simulink model "TV_2018_HIL"  (R2016a)
settings: Solver=FixedStepAuto  StartTime=0.0  StopTime=inf  FixedStep=0.001  RelTol=1e-3
PreLoadFcn:
  | TV_2017_parameters
values from neighbouring files (symbols this model uses):
  battery_voltage = single(530)    [HIL_parameters.m]    (also in HIL_parameters_2018.m; TV_2017_parameters.m; TV_2017_parameters_VD.m)
  car_params = Simulink_Car_params    [HIL_parameters.m]    (also in HIL_parameters_2018.m; TV_2017_parameters.m; TV_2017_parameters_VD.m)
  i_Diff = 16    [HIL_parameters.m]    (also in HIL_parameters_2018.m; TV_2017_parameters.m)
  Kp = 1    [HIL_parameters.m]    (also in HIL_parameters_2018.m; TV_2017_parameters.m; TV_2017_parameters_VD.m)
  motor_data = struct    [HIL_parameters.m]    (also in HIL_parameters_2018.m; TV_2017_parameters.m)
  powerLimitControl = Simulink_el    [HIL_parameters.m]    (also in HIL_parameters_2018.m; TV_2017_parameters.m; TV_2017_parameters_VD.m)
  settings = Simulink_Settings    [HIL_parameters.m]    (also in HIL_parameters_2018.m; TV_2017_parameters.m; TV_2017_parameters_VD.m)
  SpdC_BCC = 0    [HIL_parameters.m]    (also in HIL_parameters_2018.m; TV_2017_parameters.m; TV_2017_parameters_VD.m)
  Speed_Neg_sat = -21    [HIL_parameters.m]    (also in HIL_parameters_2018.m; TV_2017_parameters.m; TV_2017_parameters_VD.m)
  Speed_Pos_sat = 21    [HIL_parameters.m]    (also in HIL_parameters_2018.m; TV_2017_parameters.m; TV_2017_parameters_VD.m)
  SteeringAngleFL = [-23.80 -22.65 -21.50 -20.34 -19.18 -18.03 -16.86 -15.70 -14.53 -13.35 -12.18 -10.99 -9.80 -8.61 -7.40 -6.19 -4.97 -3.75 -2.51 -1.26 0 1.27 2.56 3.85 5.17 6.50 7.84 9.21 10.59 12.00 13.42 14.88 16.36 17.87 19.41 20.99 22.61 24.26 25.97 27.73 29.54]    [CarSetupAnalysis2018.m]    (also in HIL_parameters_2018.m; TV_2017_parameters.m; TV_2017_parameters_VD.m = [-24.129 -22.950 -21.772 -20.593 -19.413 -18.232 -17.050 -15)
  SteeringAngleFR = [-29.54 -27.73 -25.97 -24.26 -22.61 -20.99 -19.41 -17.87 -16.36 -14.88 -13.42 -12.00 -10.59 -9.21 -7.84 -6.50 -5.17 -3.85 -2.56 -1.27 0 1.26 2.51 3.75 4.97 6.19 7.40 8.61 9.80 10.99 12.18 13.35 14.53 15.70 16.86 18.03 19.18 20.34 21.50 22.65 23.80]    [CarSetupAnalysis2018.m]    (also in HIL_parameters_2018.m; TV_2017_parameters.m; TV_2017_parameters_VD.m = [-29.3050 -27.5340 -25.8140 -24.1410 -22.5110 -20.9180 -19.3)
  SteeringWhAngle = [-105 -99.75 -94.5 -89.25 -84 -78.75 -73.5 -68.25 -63 -57.75 -52.5 -47.25 -42 -36.75 -31.5 -26.25 -21.0 -15.75 -10.5 -5.25 0.0 5.25 10.50 15.75 21.00 26.25 31.50 36.75 42.00 47.25 52.50 57.75  63.00 68.25 73.50 78.75 84.00 89.25 94.50 99.75 105.00]    [TV_2017_parameters_VD.m]
  Tn_n = 0    [HIL_parameters.m]    (also in HIL_parameters_2018.m; TV_2017_parameters.m; TV_2017_parameters_VD.m)
  tractionControl = Simulink_tc    [HIL_parameters.m]    (also in HIL_parameters_2018.m; IterativeTractionControlTuning.m; TV_2017_parameters.m; TV_2017_parameters_VD.m)
  yawMomentGenerator = struct    [HIL_parameters.m]    (also in HIL_parameters_2018.m = Simulink_yawRate2; TV_2017_parameters.m = Simulink_yawRate2)
  yawRateControl = Simulink_yawRate    [HIL_parameters.m]    (also in HIL_parameters_2018.m; TV_2017_parameters.m; TV_2017_parameters_VD.m)
undefined symbols (not defined in the file or in its folder): canChannel, DiscIntNeverNeededParam, magnitude, speedEstimation, TC_Decr_Gas, TC_Derivative, TC_Incr_Gas, TC_On, TC_Relay_Off, TC_Relay_On
libraries: CarMaker4SL x366, simulink_extras x63, canmsglib x55, canlib x41, simulink x37, dspfdesign x2, sldrtlib x1
(part 5 of 15)

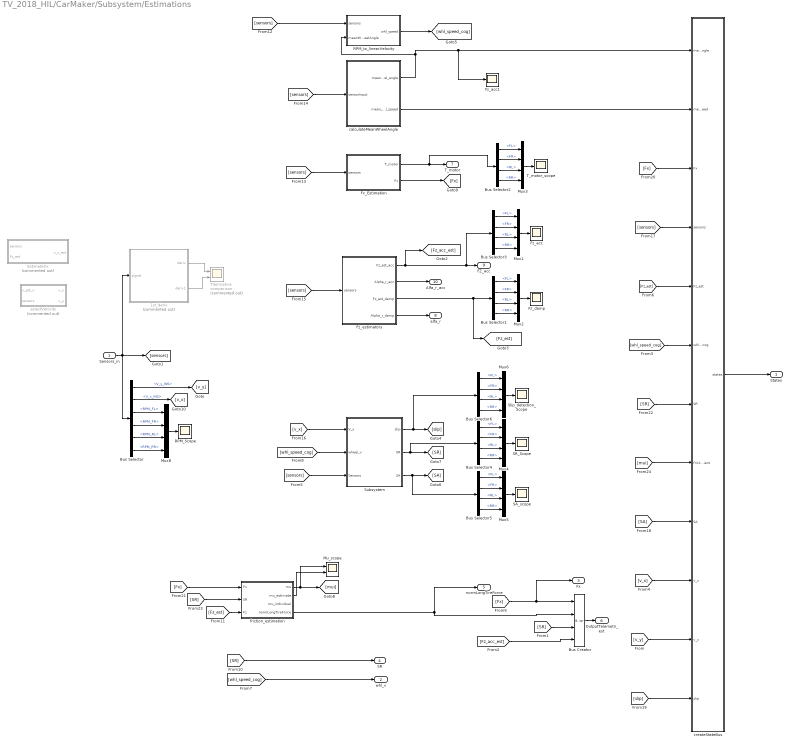
== system TV_2018_HIL/CarMaker/Subsystem/Estimations ==
  Sensors_in : Inport
  1st_deriv : Subsystem  Commented=on
  Bus Creator : BusCreator  Inputs=4  OutDataTypeStr=Bus: OutputTelemetri_est
      settings: InheritFromInputs=off
  Bus Selector : BusSelector  OutputSignals=V_y_INS,V_x_INS,RPM_FL,RPM_FR,RPM_RL,RPM_RR
  Bus Selector{1..6} (6 alike) : BusSelector  OutputSignals=FL,FR,RL,RR
  EstimateVx : Subsystem  Commented=on
  Fx_Estimation : Subsystem
  Fz_acc : Scope
  Fz_acc1 : Scope
  Fz_damp : Scope
  Fz_estimators : Subsystem
  Mu_scope : Scope  NumInputPorts=2
  Mux{1..6,8} (7 alike) : Mux
  RPM_Scope : Scope
  RPM_to_linearVelocity : Subsystem
  SA_scope : Scope
  SR_Scope : Scope
  Slip_detection_Scope : Scope
  Subsystem : Subsystem
  T_motor_scope : Scope
  Tderivative comparison : Scope  Commented=on  NumInputPorts=2
  calculateMeanWheelAngle : Subsystem
  createStateBus : Subsystem
  friction_estimation : Subsystem
  selectVelocity : Subsystem  Commented=on
  States : Outport
  whl_v : Outport  Port=2
  Fx : Outport  Port=3
  SR : Outport  Port=4
  normLongTireForce : Outport  Port=5
  OutputTelemetri_est : Outport  Port=6
  T_motor : Outport  Port=7
  alfa_r : Outport  Port=8
  FZ_acc : Outport  Port=9
  "Alfa_r_acc " : Outport  Port=10
  wires:
  Fx_Estimation/2(Fx) -> [Fx]
  RPM_to_linearVelocity/1(whl_speed) -> [whl_speed_cog]
  createStateBus/1(states) -> States/1
  [v_y] -> createStateBus/11(v_y)
  [v_x] -> createStateBus/10(v_x)
  [whl_speed_cog] -> createStateBus/6(whl_speed_cog)
  friction_estimation/1(mu) -> [mui], Mu_scope/1
  [whl_speed_cog] -> whl_v/1
  [Fx] -> Bus Creator/1, Fx/1
  [SR] -> SR/1
  friction_estimation/4(normLongTireForce) -> normLongTireForce/1, Bus Creator/2
  Bus Creator/1 -> OutputTelemetri_est/1
  [Fz_est] -> friction_estimation/3(Fz)
  calculateMeanWheelAngle/1(mean_wheel_angle) -> Fz_acc1/1, createStateBus/1(mean_wheel_angle), RPM_to_linearVelocity/2(meanWheelAngle)
  calculateMeanWheelAngle/2(mean_wheel_speed) -> createStateBus/2(mean_wheel_speed)
  Fx_Estimation/1(T_motor) -> Bus Selector2/1, T_motor/1
  Sensors_in/1 -> Bus Selector/1, [sensors], 1st_deriv/1(signal)
  [sensors] -> RPM_to_linearVelocity/1(sensors)
  [sensors] -> Fx_Estimation/1(sensors)
  [sensors] -> calculateMeanWheelAngle/1(sensorInput)
  [sensors] -> createStateBus/4(sensors)
  Bus Selector/2 -> [v_x]  "<V_x_INS>"
  Bus Selector/1 -> [v_y]  "<V_y_INS>"
  [SR] -> Bus Creator/3
  [Fz_acc_est] -> Bus Creator/4
  [Fz_est] -> createStateBus/5(Fz_est)
  [Fx] -> createStateBus/3(Fx)
  [Fx] -> friction_estimation/1(Fx)
  [SR] -> createStateBus/7(SR)
  [SR] -> friction_estimation/2(SR)
  [mui] -> createStateBus/8(frictionCoefficient)
  Bus Selector3/1 -> Mux1/1  "<FL>"
  Bus Selector3/2 -> Mux1/2  "<FR>"
  Bus Selector3/3 -> Mux1/3  "<RL>"
  Bus Selector3/4 -> Mux1/4  "<RR>"
  Mux1/1 -> Fz_acc/1
  Bus Selector1/1 -> Mux2/1  "<FL>"
  Bus Selector1/2 -> Mux2/2  "<FR>"
  Bus Selector1/3 -> Mux2/3  "<RL>"
  Bus Selector1/4 -> Mux2/4  "<RR>"
  Mux2/1 -> Fz_damp/1
  Bus Selector2/1 -> Mux3/1  "<FL>"
  Bus Selector2/2 -> Mux3/2  "<FR>"
  Bus Selector2/3 -> Mux3/3  "<RL>"
  Bus Selector2/4 -> Mux3/4  "<RR>"
  Mux3/1 -> T_motor_scope/1
  Bus Selector4/1 -> Mux4/1  "<FL>"
  Bus Selector4/2 -> Mux4/2  "<FR>"
  Bus Selector4/3 -> Mux4/3  "<RL>"
  Bus Selector4/4 -> Mux4/4  "<RR>"
  Mux4/1 -> SR_Scope/1
  1st_deriv/1(deriv) -> Tderivative comparison/1
  1st_deriv/2(deriv1) -> Tderivative comparison/2
  friction_estimation/2(mu_estimate) -> Mu_scope/2
  Bus Selector5/1 -> Mux5/1  "<FL>"
  Bus Selector5/2 -> Mux5/2  "<FR>"
  Bus Selector5/3 -> Mux5/3  "<RL>"
  Bus Selector5/4 -> Mux5/4  "<RR>"
  Mux5/1 -> SA_scope/1
  Bus Selector6/1 -> Mux6/1  "<FL>"
  Bus Selector6/2 -> Mux6/2  "<FR>"
  Bus Selector6/3 -> Mux6/3  "<RL>"
  Bus Selector6/4 -> Mux6/4  "<RR>"
  Mux6/1 -> Slip_detection_Scope/1
  Fz_estimators/3(Fz_est_damp) -> Bus Selector1/1, [Fz_est]
  Fz_estimators/1(Fz_est_acc) -> [Fz_acc_est], Bus Selector3/1, FZ_acc/1
  [sensors] -> Fz_estimators/1(sensors)
  Fz_estimators/2(Alpha_r_acc) -> "Alfa_r_acc "/1
  Fz_estimators/4(Alpha_r_damp) -> alfa_r/1
  [v_x] -> Subsystem/1(V_x)
  [whl_speed_cog] -> Subsystem/2(wheel_v)
  [sensors] -> Subsystem/3(Sensors)
  Subsystem/1(slip) -> Bus Selector6/1, [slip]
  Subsystem/2(SR) -> Bus Selector4/1, [SR]
  [SA] -> createStateBus/9(SA)
  Subsystem/3(SA) -> Bus Selector5/1, [SA]
  [slip] -> createStateBus/12(slip)
  Mux8/1 -> RPM_Scope/1
  Bus Selector/3 -> Mux8/1  "<RPM_FL>"
  Bus Selector/4 -> Mux8/2  "<RPM_FR>"
  Bus Selector/5 -> Mux8/3  "<RPM_RL>"
  Bus Selector/6 -> Mux8/4  "<RPM_RR>"

== system TV_2018_HIL/CarMaker/VehicleControl3/CreateBus Vhcl.Misc ==
  In1 : Inport
  BusCreator : BusCreator  Inputs=11
  Demux : Demux  Outputs=11
  Out1 : Outport
  wires:
  Demux/11 -> BusCreator/11  "Vhcl Wind_vel_0 z"
  Demux/10 -> BusCreator/10  "Vhcl Wind_vel_0 y"
  Demux/9 -> BusCreator/9  "Vhcl Wind_vel_0 x"
  Demux/8 -> BusCreator/8  "Vhcl Trq_DL2BdyEng y"
  Demux/7 -> BusCreator/7  "Vhcl Trq_DL2BdyEng x"
  Demux/6 -> BusCreator/6  "Vhcl Trq_DL2Bdy1B z"
  Demux/5 -> BusCreator/5  "Vhcl Trq_DL2Bdy1B y"
  Demux/4 -> BusCreator/4  "Vhcl Trq_DL2Bdy1B x"
  Demux/3 -> BusCreator/3  "Vhcl Trq_DL2Bdy1 z"
  Demux/2 -> BusCreator/2  "Vhcl Trq_DL2Bdy1 y"
  Demux/1 -> BusCreator/1  "Vhcl Trq_DL2Bdy1 x"
  In1/1 -> Demux/1
  BusCreator/1 -> Out1/1

== system TV_2018_HIL/CarMaker/VehicleControl3/CreateBus Vhcl.Wheel.In ==
  In1 : Inport
  Bus Creator1 : BusCreator  Inputs=12
  Demux1 : Demux  Outputs=12
  Out1 : Outport
  wires:
  Demux1/12 -> Bus Creator1/12  "Vhcl Wheel RR rotv"
  Demux1/11 -> Bus Creator1/11  "Vhcl Wheel RR Trq_DL2WC"
  Demux1/10 -> Bus Creator1/10  "Vhcl Wheel RR Trq_B2WC"
  Demux1/9 -> Bus Creator1/9  "Vhcl Wheel RL rotv"
  Demux1/8 -> Bus Creator1/8  "Vhcl Wheel RL Trq_DL2WC"
  Demux1/7 -> Bus Creator1/7  "Vhcl Wheel RL Trq_B2WC"
  Demux1/6 -> Bus Creator1/6  "Vhcl Wheel FR rotv"
  Demux1/5 -> Bus Creator1/5  "Vhcl Wheel FR Trq_DL2WC"
  Demux1/4 -> Bus Creator1/4  "Vhcl Wheel FR Trq_B2WC"
  Demux1/3 -> Bus Creator1/3  "Vhcl Wheel FL rotv"
  In1/1 -> Demux1/1
  Bus Creator1/1 -> Out1/1
  Demux1/2 -> Bus Creator1/2  "Vhcl Wheel FL Trq_DL2WC"
  Demux1/1 -> Bus Creator1/1  "Vhcl Wheel FL Trq_B2WC"

== system TV_2018_HIL/CarMaker/VehicleControl3/CreateBus VhclCtrl ==
  In : Inport
  BusCreator : BusCreator  Inputs=29
  Demux : Demux  Outputs=29
  Out : Outport
  wires:
  In/1 -> Demux/1
  BusCreator/1 -> Out/1
  Demux/1 -> BusCreator/1  "VhclCtrl SST"
  Demux/2 -> BusCreator/2  "VhclCtrl Key"
  Demux/3 -> BusCreator/3  "VhclCtrl UserSignal0"
  Demux/4 -> BusCreator/4  "VhclCtrl UserSignal1"
  Demux/5 -> BusCreator/5  "VhclCtrl UserSignal2"
  Demux/6 -> BusCreator/6  "VhclCtrl UserSignal3"
  Demux/7 -> BusCreator/7  "VhclCtrl UserSignal4"
  Demux/8 -> BusCreator/8  "VhclCtrl GearNo"
  Demux/9 -> BusCreator/9  "VhclCtrl SelectorCtrl"
  Demux/10 -> BusCreator/10  "VhclCtrl Brake"
  Demux/11 -> BusCreator/11  "VhclCtrl BrakePark"
  Demux/12 -> BusCreator/12  "VhclCtrl Clutch"
  Demux/13 -> BusCreator/13  "VhclCtrl Gas"
  Demux/14 -> BusCreator/14  "VhclCtrl Steering Ang"
  Demux/15 -> BusCreator/15  "VhclCtrl Steering AngVel"
  Demux/16 -> BusCreator/16  "VhclCtrl Steering AngAcc"
  Demux/17 -> BusCreator/17  "VhclCtrl Steering Trq"
  Demux/18 -> BusCreator/18  "VhclCtrl Lights LowBeam"
  Demux/19 -> BusCreator/19  "VhclCtrl Lights HighBeam"
  Demux/20 -> BusCreator/20  "VhclCtrl Lights Daytime"
  Demux/21 -> BusCreator/21  "VhclCtrl Lights ParkL"
  Demux/22 -> BusCreator/22  "VhclCtrl Lights ParkR"
  Demux/23 -> BusCreator/23  "VhclCtrl Lights IndL"
  Demux/24 -> BusCreator/24  "VhclCtrl Lights IndR"
  Demux/25 -> BusCreator/25  "VhclCtrl Lights FogFrontL"
  Demux/26 -> BusCreator/26  "VhclCtrl Lights FogFrontR"
  Demux/27 -> BusCreator/27  "VhclCtrl Lights FogRear"
  Demux/28 -> BusCreator/28  "VhclCtrl Lights Brake"
  Demux/29 -> BusCreator/29  "VhclCtrl Lights Reverse"

== system TV_2018_HIL/CarMaker/VehicleControl3/CreateBus VhclCtrl.PT ==
  In1 : Inport
  BusCreator1 : BusCreator  Inputs=12
  Demux1 : Demux  Outputs=12
  Out1 : Outport
  wires:
  Demux1/12 -> BusCreator1/12  "VhclCtrl Brake"
  Demux1/11 -> BusCreator1/11  "VhclCtrl Gas"
  Demux1/10 -> BusCreator1/10  "VhclCtrl Clutch"
  Demux1/9 -> BusCreator1/9  "VhclCtrl SelectorCtrl"
  Demux1/8 -> BusCreator1/8  "VhclCtrl GearNo"
  Demux1/7 -> BusCreator1/7  "VhclCtrl UserSignal4"
  Demux1/6 -> BusCreator1/6  "VhclCtrl UserSignal3"
  Demux1/5 -> BusCreator1/5  "VhclCtrl UserSignal2"
  Demux1/4 -> BusCreator1/4  "VhclCtrl UserSignal1"
  Demux1/3 -> BusCreator1/3  "VhclCtrl UserSignal0"
  Demux1/2 -> BusCreator1/2  "VhclCtrl Key"
  Demux1/1 -> BusCreator1/1  "VhclCtrl SST"
  In1/1 -> Demux1/1
  BusCreator1/1 -> Out1/1

== system TV_2018_HIL/CarMaker/VehicleControl3/CreateBus VhclCtrl.Steering ==
  In1 : Inport
  Bus Creator : BusCreator  Inputs=5
  Demux : Demux  Outputs=5
  Out1 : Outport
  wires:
  In1/1 -> Demux/1
  Bus Creator/1 -> Out1/1
  Demux/1 -> Bus Creator/1  "VhclCtrl Steering Ang"
  Demux/5 -> Bus Creator/5  "VhclCtrl Steering SteerByTrq"
  Demux/3 -> Bus Creator/3  "VhclCtrl Steering AngAcc"
  Demux/2 -> Bus Creator/2  "VhclCtrl Steering AngVel"
  Demux/4 -> Bus Creator/4  "VhclCtrl Steering Trq"

== system TV_2018_HIL/CarMaker/IPG Vehicle3/Brake/CreateBus Vhcl.Wheel.PT ==
  In : Inport
  BusCreator1 : BusCreator  Inputs=20
  Demux1 : Demux  Outputs=20
  Out : Outport
  wires:
  Demux1/20 -> BusCreator1/20  "Vhcl Trq_DriveSrc_trg d3"
  Demux1/19 -> BusCreator1/19  "Vhcl Trq_DriveSrc_trg d2"
  Demux1/18 -> BusCreator1/18  "Vhcl Trq_DriveSrc_trg d1"
  Demux1/17 -> BusCreator1/17  "Vhcl Trq_DriveSrc_trg d0"
  Demux1/16 -> BusCreator1/16  "Vhcl Wheel RR WhlBearing"
  Demux1/15 -> BusCreator1/15  "Vhcl Wheel RR Trq_T2W"
  Demux1/14 -> BusCreator1/14  "Vhcl Wheel RR Trq_BrakeReg_trg"
  Demux1/13 -> BusCreator1/13  "Vhcl Wheel RR Trq_Brake"
  Demux1/12 -> BusCreator1/12  "Vhcl Wheel RL WhlBearing"
  Demux1/11 -> BusCreator1/11  "Vhcl Wheel RL Trq_T2W"
  Demux1/10 -> BusCreator1/10  "Vhcl Wheel RL Trq_BrakeReg_trg"
  Demux1/9 -> BusCreator1/9  "Vhcl Wheel RL Trq_Brake"
  Demux1/8 -> BusCreator1/8  "Vhcl Wheel FR WhlBearing"
  Demux1/7 -> BusCreator1/7  "Vhcl Wheel FR Trq_T2W"
  Demux1/6 -> BusCreator1/6  "Vhcl Wheel FR Trq_BrakeReg_trg"
  Demux1/5 -> BusCreator1/5  "Vhcl Wheel FR Trq_Brake"
  Demux1/4 -> BusCreator1/4  "Vhcl Wheel FL WhlBearing"
  Demux1/3 -> BusCreator1/3  "Vhcl Wheel FL Trq_T2W"
  Demux1/2 -> BusCreator1/2  "Vhcl Wheel FL Trq_BrakeReg_trg"
  Demux1/1 -> BusCreator1/1  "Vhcl Wheel FL Trq_Brake"
  BusCreator1/1 -> Out/1
  In/1 -> Demux1/1

== system TV_2018_HIL/CarMaker/IPG Vehicle3/CarAndTrailer/CarAndTrailerUpd ==
  Sync_In : Inport
  Vhcl.Steering : Inport  Port=2
  Vhcl.Motion : Inport  Port=3
  Vhcl.PoI : Inport  Port=4
  Vhcl.Wheel.FL : Inport  Port=5
  Vhcl.Wheel.FR : Inport  Port=6
  Vhcl.Wheel.RL : Inport  Port=7
  Vhcl.Wheel.RR : Inport  Port=8
  Car.Hitch.FrcTrq : Inport  Port=9
  Vhcl.Fr1A : Inport  Port=10
  CarAndTrailerUpd : S-Function  FunctionName=CM_Sfun  Parameters='CarAndTrUpd'  SFunctionDeploymentMode=off  EnableBusSupport=off
  CreateBus Brake.IF.In : Subsystem
  Sync_Out : Outport
  Brake.IF.In : Outport  Port=2
  wires:
  Vhcl.Fr1A/1 -> CarAndTrailerUpd/10  "user vehicle only"
  Vhcl.Steering/1 -> CarAndTrailerUpd/2
  Vhcl.Motion/1 -> CarAndTrailerUpd/3
  Vhcl.PoI/1 -> CarAndTrailerUpd/4
  Vhcl.Wheel.FL/1 -> CarAndTrailerUpd/5
  Vhcl.Wheel.FR/1 -> CarAndTrailerUpd/6
  Car.Hitch.FrcTrq/1 -> CarAndTrailerUpd/9
  Vhcl.Wheel.RR/1 -> CarAndTrailerUpd/8
  Vhcl.Wheel.RL/1 -> CarAndTrailerUpd/7
  CarAndTrailerUpd/2 -> CreateBus Brake.IF.In/1(In)
  CreateBus Brake.IF.In/1(Out) -> Brake.IF.In/1
  CarAndTrailerUpd/1 -> Sync_Out/1
  Sync_In/1 -> CarAndTrailerUpd/1

== system TV_2018_HIL/CarMaker/IPG Vehicle3/CarAndTrailer/Forces ==
  Sync_In : Inport
  TireFL_In : Inport  Port=2
  TireFR_In : Inport  Port=3
  TireRL_In : Inport  Port=4
  TireRR_In : Inport  Port=5
  lSpring : Inport  Port=6
  vDamp : Inport  Port=7
  lStabi : Inport  Port=8
  lBuf : Inport  Port=9
  External Suspension Forces : Subsystem
  Tires : Subsystem
  Vehicle Forces : Subsystem
  Sync_Out : Outport
  Car.Virtual : Outport  Port=2
  Car.Aero : Outport  Port=3
  Car.Load : Outport  Port=4
  TireFL_Out : Outport  Port=5
  TireFR_Out : Outport  Port=6
  TireRL_Out : Outport  Port=7
  TireRR_Out : Outport  Port=8
  FSpring : Outport  Port=9
  FDamp : Outport  Port=10
  FStabi : Outport  Port=11
  FBuf : Outport  Port=12
  wires:
  lBuf/1 -> External Suspension Forces/5(lBuf)
  lStabi/1 -> External Suspension Forces/4(lStabi)
  vDamp/1 -> External Suspension Forces/3(vDamp)
  Tires/4(TireRR_Out) -> TireRR_Out/1
  Tires/3(TireRL_Out) -> TireRL_Out/1
  Tires/2(TireFR_Out) -> TireFR_Out/1
  Tires/1(TireFL_Out) -> TireFL_Out/1
  TireRR_In/1 -> Tires/5(TireRR_In)
  TireRL_In/1 -> Tires/4(TireRL_In)
  TireFR_In/1 -> Tires/3(TireFR_In)
  TireFL_In/1 -> Tires/2(TireFL_In)
  External Suspension Forces/4(FBuf) -> FBuf/1
  Sync_In/1 -> External Suspension Forces/1(Sync_In), Tires/1(Sync_In), Vehicle Forces/1(Sync_In)
  Vehicle Forces/1(Sync_Out) -> Sync_Out/1
  Vehicle Forces/2(Car.Virtual) -> Car.Virtual/1
  Vehicle Forces/3(Car.Aero) -> Car.Aero/1
  Vehicle Forces/4(Car.Load) -> Car.Load/1
  lSpring/1 -> External Suspension Forces/2(lSpring)
  External Suspension Forces/2(FDamp) -> FDamp/1
  External Suspension Forces/3(FStabi) -> FStabi/1
  External Suspension Forces/1(FSpring) -> FSpring/1

== system TV_2018_HIL/CarMaker/IPG Vehicle3/CarAndTrailer/Kinematics ==
  Sync_In : Inport
  Steer.IF : Inport  Port=2
  Kinematics : S-Function  FunctionName=CM_Sfun  Parameters='Kinematics'  SFunctionDeploymentMode=off  EnableBusSupport=off
  Sync_Out : Outport
  TireFL_In : Outport  Port=2
  TireFR_In : Outport  Port=3
  TireRL_In : Outport  Port=4
  TireRR_In : Outport  Port=5
  lSpring : Outport  Port=6
  vDamp : Outport  Port=7
  lStabi : Outport  Port=8
  lBuf : Outport  Port=9
  wires:
  Kinematics/9 -> lBuf/1
  Kinematics/8 -> lStabi/1
  Kinematics/2 -> TireFL_In/1
  Kinematics/3 -> TireFR_In/1
  Kinematics/4 -> TireRL_In/1
  Kinematics/5 -> TireRR_In/1
  Kinematics/6 -> lSpring/1
  Kinematics/7 -> vDamp/1
  Sync_In/1 -> Kinematics/1
  Kinematics/1 -> Sync_Out/1
  Steer.IF/1 -> Kinematics/2

== system TV_2018_HIL/CarMaker/IPG Vehicle3/CarAndTrailer/Kinetics ==
  Sync_In : Inport
  Car.Virtual : Inport  Port=2
  Car.Aero : Inport  Port=3
  Car.Load : Inport  Port=4
  TireFL.Out : Inport  Port=5
  TireFR.Out : Inport  Port=6
  TireRL.Out : Inport  Port=7
  TireRR.Out : Inport  Port=8
  FSpring : Inport  Port=9
  FDamp : Inport  Port=10
  FStabi : Inport  Port=11
  FBuf : Inport  Port=12
  Bus Creator : BusCreator  Inputs=4
  Bus Creator1 : BusCreator  Inputs=12
  Bus Creator2 : BusCreator  Inputs=6
  Bus Creator3 : BusCreator  Inputs=6
  Bus Creator4 : BusCreator  Inputs=4
  Demux : Demux  Outputs=12
  Demux1 : Demux  Outputs=6
  Demux2 : Demux  Outputs=6
  Demux3 : Demux
  Demux4 : Demux
  Kinetics : S-Function  FunctionName=CM_Sfun  Parameters='Kinetics'  SFunctionDeploymentMode=off  EnableBusSupport=off
  Sync_Out : Outport
  Trailer.Load : Outport  Port=2
  Car.Hitch : Outport  Port=3
  Car.Fr1 : Outport  Port=4
  Car.Trq_T2W : Outport  Port=5
  WheelCarrier.Misc : Outport  Port=6
  wires:
  FBuf/1 -> Kinetics/12
  Sync_In/1 -> Kinetics/1
  Kinetics/1 -> Sync_Out/1
  Car.Aero/1 -> Kinetics/3
  Car.Virtual/1 -> Kinetics/2
  Bus Creator1/1 -> Trailer.Load/1
  Demux/1 -> Bus Creator1/1  "Trailer Load_0 mass"
  Demux/2 -> Bus Creator1/2  "Trailer Load_0 tx"
  Demux/3 -> Bus Creator1/3  "Trailer Load_0 ty"
  Demux/4 -> Bus Creator1/4  "Trailer Load_0 tz"
  Kinetics/2 -> Demux/1
  Demux/5 -> Bus Creator1/5  "Trailer Load_1 mass"
  Demux/6 -> Bus Creator1/6  "Trailer Load_1 tx"
  Demux/7 -> Bus Creator1/7  "Trailer Load_1 ty"
  Demux/8 -> Bus Creator1/8  "Trailer Load_1 tz"
  Demux/9 -> Bus Creator1/9  "Trailer Load_2 mass"
  Demux/10 -> Bus Creator1/10  "Trailer Load_2 tx"
  Demux/11 -> Bus Creator1/11  "Trailer Load_2 ty"
  Demux/12 -> Bus Creator1/12  "Trailer Load_2 tz"
  Demux1/1 -> Bus Creator2/1  "Car Hitch tx"
  Demux1/2 -> Bus Creator2/2  "Car Hitch ty"
  Demux1/3 -> Bus Creator2/3  "Car Hitch tz"
  Demux1/4 -> Bus Creator2/4  "Car Hitch vx"
  Demux1/5 -> Bus Creator2/5  "Car Hitch vy"
  Demux1/6 -> Bus Creator2/6  "Car Hitch vz"
  Kinetics/3 -> Demux1/1
  Bus Creator2/1 -> Car.Hitch/1
  Demux2/1 -> Bus Creator3/1  "Car Fr1 rx"
  Demux2/2 -> Bus Creator3/2  "Car Fr1 ry"
  Demux2/3 -> Bus Creator3/3  "Car Fr1 rz"
  Demux2/4 -> Bus Creator3/4  "Car Fr1 rvx"
  Demux2/5 -> Bus Creator3/5  "Car Fr1 rvy"
  Demux2/6 -> Bus Creator3/6  "Car Fr1 rvz"
  Bus Creator3/1 -> Car.Fr1/1
  Kinetics/4 -> Demux2/1
  Car.Load/1 -> Kinetics/4
  Demux3/1 -> Bus Creator4/1  "car Susp FL GenInert2"
  Demux3/2 -> Bus Creator4/2  "car Susp FR GenInert2"
  Demux3/3 -> Bus Creator4/3  "car Susp FL GenFrc2"
  Demux3/4 -> Bus Creator4/4  "car Susp FR GenFrc2"
  Bus Creator4/1 -> WheelCarrier.Misc/1
  Bus Creator/1 -> Car.Trq_T2W/1
  Demux4/4 -> Bus Creator/4  "Car Trq_T2WRR"
  Demux4/3 -> Bus Creator/3  "Car Trq_T2WRL"
  Demux4/2 -> Bus Creator/2  "Car Trq_T2WFR"
  Demux4/1 -> Bus Creator/1  "Car Trq_T2WFL"
  TireFL.Out/1 -> Kinetics/5
  TireFR.Out/1 -> Kinetics/6
  TireRL.Out/1 -> Kinetics/7
  TireRR.Out/1 -> Kinetics/8
  FSpring/1 -> Kinetics/9
  FDamp/1 -> Kinetics/10
  FStabi/1 -> Kinetics/11
  Kinetics/6 -> Demux3/1
  Kinetics/5 -> Demux4/1

== system TV_2018_HIL/CarMaker/IPG Vehicle3/CarAndTrailer/Steering ==
  note: When replacing the entire steering system,
      | be sure to add '-disablesteering' to the command line arguments
      | in the CarMaker Model Configuration block.
  Sync_In : Inport
  VhclCtrl.Steering : Inport  Port=2
  Bus Creator1 : BusCreator  Inputs=16
  Bus Creator2 : BusCreator  Inputs=5
  Demux : Demux  Outputs=21
  Steering : S-Function  FunctionName=CM_Sfun  Parameters='Steering'  SFunctionDeploymentMode=off  EnableBusSupport=off
  Terminator : Terminator
  Sync_Out : Outport
  Steer.IF : Outport  Port=2
  wires:
  Demux/21 -> Bus Creator2/5  "Steering IF R Inert"
  Demux/20 -> Bus Creator2/4  "Steering IF R Frc"
  Demux/19 -> Bus Creator2/3  "Steering IF L Inert"
  Demux/18 -> Bus Creator2/2  "Steering IF L Frc"
  Demux/17 -> Bus Creator2/1  "Steering IF SteerByTrq"
  Demux/16 -> Bus Creator1/16  "Steering IF R iSteer2q"
  Demux/15 -> Bus Creator1/15  "Steering IF R qpp"
  Demux/14 -> Bus Creator1/14  "Steering IF R qp"
  Demux/13 -> Bus Creator1/13  "Steering IF R q"
  Demux/12 -> Bus Creator1/12  "Steering IF L iSteer2q"
  Demux/11 -> Bus Creator1/11  "Steering IF L qpp"
  Demux/10 -> Bus Creator1/10  "Steering IF L qp"
  Demux/9 -> Bus Creator1/9  "Steering IF L q"
  Demux/8 -> Bus Creator1/8  "Steering IF AssistTrqPin"
  Demux/7 -> Bus Creator1/7  "Steering IF AssistTrqCol"
  Demux/6 -> Bus Creator1/6  "Steering IF AssistFrc"
  Demux/5 -> Bus Creator1/5  "Steering IF TrqStatic"
  Demux/4 -> Bus Creator1/4  "Steering IF Trq"
  Demux/3 -> Bus Creator1/3  "Steering IF AngAcc"
  Demux/2 -> Bus Creator1/2  "Steering IF AngVel"
  Demux/1 -> Bus Creator1/1  "Steering IF Ang"
  Bus Creator1/1 -> Steer.IF/1
  Steering/2 -> Demux/1
  Bus Creator2/1 -> Terminator/1  "Steer IF (in)"
  VhclCtrl.Steering/1 -> Steering/2
  Steering/1 -> Sync_Out/1
  Sync_In/1 -> Steering/1

== system TV_2018_HIL/CarMaker/IPG Vehicle3/CarAndTrailer/Trailer ==
  Sync_In : Inport
  Trailer.Load : Inport  Port=2
  Car.Hitch : Inport  Port=3
  Car.Fr1 : Inport  Port=4
  Car.Trq_T2W : Inport  Port=5
  WheelCarrier.Misc : Inport  Port=6
  CreateBus Car.Hitch.FrcTrq : Subsystem
  CreateBus Vhcl.Motion : Subsystem
  CreateBus Vhcl.PoI : Subsystem
  CreateBus Vhcl.Steering : Subsystem
  CreateBus Vhcl.Wheel.FL : Subsystem
  CreateBus Vhcl.Wheel.FR : Subsystem
  CreateBus Vhcl.Wheel.RL : Subsystem
  CreateBus Vhcl.Wheel.RR : Subsystem
  Trailer : S-Function  FunctionName=CM_Sfun  Parameters='Trailer'  SFunctionDeploymentMode=off  EnableBusSupport=off
  Sync_Out : Outport
  Vhcl.Steering : Outport  Port=2
  Vhcl.Motion : Outport  Port=3
  Vhcl.PoI : Outport  Port=4
  Vhcl.Wheel.FL : Outport  Port=5
  Vhcl.Wheel.FR : Outport  Port=6
  Vhcl.Wheel.RL : Outport  Port=7
  Vhcl.Wheel.RR : Outport  Port=8
  Car.Hitch.FrcTrq : Outport  Port=9
  wires:
  Trailer/2 -> CreateBus Vhcl.Steering/1(In1)
  CreateBus Vhcl.Steering/1(Out1) -> Vhcl.Steering/1  "Vhcl.Steering"
  Trailer/3 -> CreateBus Vhcl.Motion/1(In1)
  Trailer/4 -> CreateBus Vhcl.PoI/1(In1)
  Trailer/5 -> CreateBus Vhcl.Wheel.FL/1(In1)
  Trailer/6 -> CreateBus Vhcl.Wheel.FR/1(In1)
  Trailer/7 -> CreateBus Vhcl.Wheel.RL/1(In1)
  Trailer/9 -> CreateBus Car.Hitch.FrcTrq/1(In1)
  Trailer/8 -> CreateBus Vhcl.Wheel.RR/1(In1)
  CreateBus Vhcl.Wheel.RR/1(Out1) -> Vhcl.Wheel.RR/1  "Vhcl.Wheel.RR"
  CreateBus Vhcl.Wheel.RL/1(Out1) -> Vhcl.Wheel.RL/1  "Vhcl.Wheel.RL"
  CreateBus Vhcl.Wheel.FR/1(Out1) -> Vhcl.Wheel.FR/1  "Vhcl.Wheel.FR"
  CreateBus Vhcl.Wheel.FL/1(Out1) -> Vhcl.Wheel.FL/1  "Vhcl.Wheel.FL"
  CreateBus Vhcl.PoI/1(Out1) -> Vhcl.PoI/1  "Vhcl.PoI"
  CreateBus Vhcl.Motion/1(Out1) -> Vhcl.Motion/1  "Vhcl.Motion"
  Car.Trq_T2W/1 -> Trailer/5
  WheelCarrier.Misc/1 -> Trailer/6
  CreateBus Car.Hitch.FrcTrq/1(Out1) -> Car.Hitch.FrcTrq/1  "Car.Hitch.FrcTrq"
  Car.Fr1/1 -> Trailer/4
  Car.Hitch/1 -> Trailer/3
  Trailer.Load/1 -> Trailer/2
  Trailer/1 -> Sync_Out/1
  Sync_In/1 -> Trailer/1

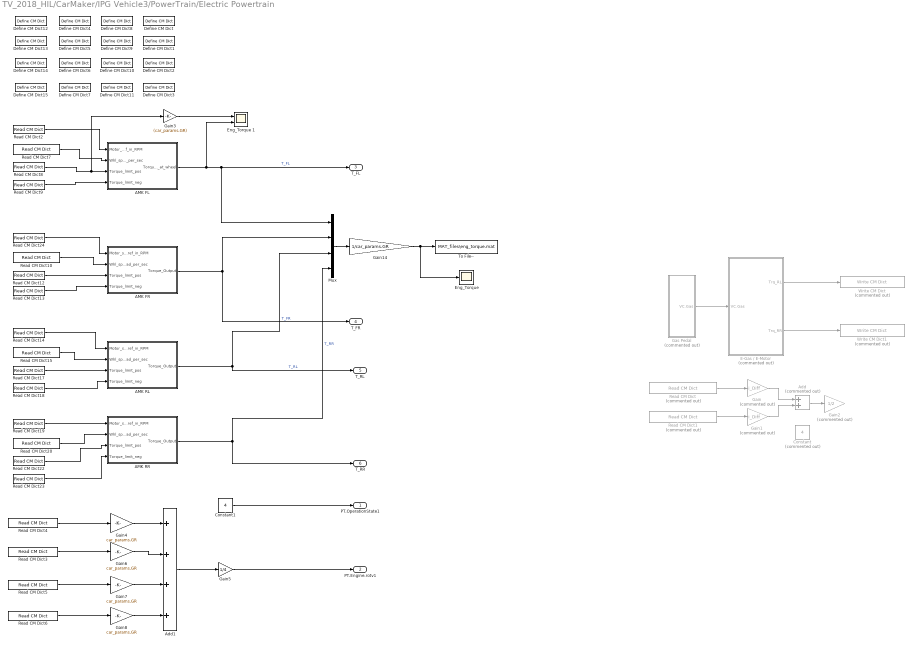
== system TV_2018_HIL/CarMaker/IPG Vehicle3/PowerTrain/Electric Powertrain ==
  AMK FL : Subsystem
  AMK FR : Subsystem
  AMK RL : Subsystem
  AMK RR : Subsystem
  Add : Sum  Commented=on
  Add1 : Sum  Inputs=++++
  Constant : Constant  Commented=on  Value=4
  Constant1 : Constant  Value=4
  Define CM Dict : CarMaker4SL/Define CM Dict  xname=T_req_RL  xmono=off  xtype=Double4  xdvaplace=None  xnstates=0  xfirststate=0  xinitial=0
  Define CM Dict1 : CarMaker4SL/Define CM Dict  xname=T_req_RR  xmono=off  xtype=Double4  xdvaplace=None  xnstates=0  xfirststate=0  xinitial=0
  Define CM Dict10 : CarMaker4SL/Define CM Dict  xname=Tlim_neg_RL  xmono=off  xtype=Double4  xdvaplace=None  xnstates=0  xfirststate=0  xinitial=0
  Define CM Dict11 : CarMaker4SL/Define CM Dict  xname=Tlim_neg_RR  xmono=off  xtype=Double4  xdvaplace=None  xnstates=0  xfirststate=0  xinitial=0
  Define CM Dict12 : CarMaker4SL/Define CM Dict  xname=w_set_FL  xmono=off  xtype=Double4  xdvaplace=None  xnstates=0  xfirststate=0  xinitial=0
  Define CM Dict13 : CarMaker4SL/Define CM Dict  xname=w_set_FR  xmono=off  xtype=Double4  xdvaplace=None  xnstates=0  xfirststate=0  xinitial=0
  Define CM Dict14 : CarMaker4SL/Define CM Dict  xname=w_set_RL  xmono=off  xtype=Double4  xdvaplace=None  xnstates=0  xfirststate=0  xinitial=0
  Define CM Dict15 : CarMaker4SL/Define CM Dict  xname=w_set_RR  xmono=off  xtype=Double4  xdvaplace=None  xnstates=0  xfirststate=0  xinitial=0
  Define CM Dict2 : CarMaker4SL/Define CM Dict  xname=T_req_FL  xmono=off  xtype=Double4  xdvaplace=None  xnstates=0  xfirststate=0  xinitial=0
  Define CM Dict3 : CarMaker4SL/Define CM Dict  xname=T_req_FR  xmono=off  xtype=Double4  xdvaplace=None  xnstates=0  xfirststate=0  xinitial=0
  Define CM Dict4 : CarMaker4SL/Define CM Dict  xname=Tlim_pos_FL  xmono=off  xtype=Double4  xdvaplace=None  xnstates=0  xfirststate=0  xinitial=0
  Define CM Dict5 : CarMaker4SL/Define CM Dict  xname=Tlim_pos_FR  xmono=off  xtype=Double4  xdvaplace=None  xnstates=0  xfirststate=0  xinitial=0
  Define CM Dict6 : CarMaker4SL/Define CM Dict  xname=Tlim_pos_RL  xmono=off  xtype=Double4  xdvaplace=None  xnstates=0  xfirststate=0  xinitial=0
  Define CM Dict7 : CarMaker4SL/Define CM Dict  xname=Tlim_pos_RR  xmono=off  xtype=Double4  xdvaplace=None  xnstates=0  xfirststate=0  xinitial=0
  Define CM Dict8 : CarMaker4SL/Define CM Dict  xname=Tlim_neg_FL  xmono=off  xtype=Double4  xdvaplace=None  xnstates=0  xfirststate=0  xinitial=0
  Define CM Dict9 : CarMaker4SL/Define CM Dict  xname=Tlim_neg_FR  xmono=off  xtype=Double4  xdvaplace=None  xnstates=0  xfirststate=0  xinitial=0
  E-Gas / E-Motor : Subsystem  Commented=on
  "Eng_Torque " : Scope
  Eng_Torque 1 : Scope  NumInputPorts=2
  Gain : Gain  Commented=on  Gain=i_Diff
  Gain1 : Gain  Commented=on  Gain=i_Diff
  Gain14 : Gain  Gain=1/car_params.GR
  Gain2 : Gain  Commented=on  Gain=1/2
  Gain3 : Gain  Gain=(car_params.GR)
  Gain{4,6..8} (4 alike) : Gain  Gain=car_params.GR
  Gain5 : Gain  Gain=1/4
  Gas Pedal : Subsystem  Commented=on
  Mux : Mux
  Read CM Dict : CarMaker4SL/Read CM Dict  Commented=on  xname=Car.WheelSpd_RL  xsync=off
  Read CM Dict1 : CarMaker4SL/Read CM Dict  Commented=on  xname=Car.WheelSpd_RR  xsync=off
  Read CM Dict10 : CarMaker4SL/Read CM Dict  xname=Car.WheelSpd_FR  xsync=off
  Read CM Dict12 : CarMaker4SL/Read CM Dict  xname=Tlim_pos_FR  xsync=off
  Read CM Dict13 : CarMaker4SL/Read CM Dict  xname=Tlim_neg_FR  xsync=off
  Read CM Dict14 : CarMaker4SL/Read CM Dict  xname=w_set_RL  xsync=off
  Read CM Dict15 : CarMaker4SL/Read CM Dict  xname=Car.WheelSpd_RL  xsync=off
  Read CM Dict17 : CarMaker4SL/Read CM Dict  xname=Tlim_pos_RL  xsync=off
  Read CM Dict18 : CarMaker4SL/Read CM Dict  xname=Tlim_neg_RL  xsync=off
  Read CM Dict19 : CarMaker4SL/Read CM Dict  xname=w_set_RR  xsync=off
  Read CM Dict2 : CarMaker4SL/Read CM Dict  xname=w_set_FL  xsync=off
  Read CM Dict20 : CarMaker4SL/Read CM Dict  xname=Car.WheelSpd_RR  xsync=off
  Read CM Dict22 : CarMaker4SL/Read CM Dict  xname=Tlim_pos_RR  xsync=off
  Read CM Dict23 : CarMaker4SL/Read CM Dict  xname=Tlim_neg_RR  xsync=off
  Read CM Dict24 : CarMaker4SL/Read CM Dict  xname=w_set_FR  xsync=off
  Read CM Dict3 : CarMaker4SL/Read CM Dict  xname=Car.WheelSpd_RR  xsync=off
  Read CM Dict4 : CarMaker4SL/Read CM Dict  xname=Car.WheelSpd_RL  xsync=off
  Read CM Dict5 : CarMaker4SL/Read CM Dict  xname=Car.WheelSpd_FR  xsync=off
  Read CM Dict6 : CarMaker4SL/Read CM Dict  xname=Car.WheelSpd_FL  xsync=off
  Read CM Dict7 : CarMaker4SL/Read CM Dict  xname=Car.WheelSpd_FL  xsync=off
  Read CM Dict8 : CarMaker4SL/Read CM Dict  xname=Tlim_pos_FL  xsync=off
  Read CM Dict9 : CarMaker4SL/Read CM Dict  xname=Tlim_neg_FL  xsync=off
  To File-- : ToFile  Filename=MAT_files\eng_torque.mat  MatrixName=torques  SaveFormat=Timeseries
  Write CM Dict : CarMaker4SL/Write CM Dict  Commented=on  xname=PT.WRL.Trq_Drive  xsync=off
  Write CM Dict1 : CarMaker4SL/Write CM Dict  Commented=on  xname=PT.WRR.Trq_Drive  xsync=off
  PT.OperationState1 : Outport
  PT.Engine.rotv1 : Outport  Port=2
  T_FL : Outport  Port=3
  T_FR : Outport  Port=4
  T_RL : Outport  Port=5
  T_RR : Outport  Port=6
  wires:
  Gas Pedal/1(VC.Gas) -> E-Gas / E-Motor/1(VC.Gas)
  E-Gas / E-Motor/1(Trq_RL) -> Write CM Dict/1
  E-Gas / E-Motor/2(Trq_RR) -> Write CM Dict1/1
  Read CM Dict1/1 -> Gain1/1
  Read CM Dict/1 -> Gain/1
  Gain/1 -> Add/1
  Gain1/1 -> Add/2
  Add/1 -> Gain2/1
  Constant1/1 -> PT.OperationState1/1
  Gain4/1 -> Add1/1
  Gain6/1 -> Add1/2
  Add1/1 -> Gain5/1
  Gain5/1 -> PT.Engine.rotv1/1
  Gain7/1 -> Add1/3
  Gain8/1 -> Add1/4
  Read CM Dict7/1 -> AMK FL/2(Whl_speed_rad_per_sec)
  Read CM Dict9/1 -> AMK FL/4(Torque_limit_neg)
  Read CM Dict2/1 -> AMK FL/1(Motor_speed_ref_in_RPM)
  AMK FL/1("Torque_output_at_wheel ") -> Eng_Torque 1/2, T_FL/1, Mux/1  "T_FL"
  Read CM Dict10/1 -> AMK FR/2(Whl_speed_rad_per_sec)
  Read CM Dict12/1 -> AMK FR/3("Torque_limit_pos ")
  Read CM Dict13/1 -> AMK FR/4(Torque_limit_neg)
  Read CM Dict24/1 -> AMK FR/1(Motor_speed_ref_in_RPM)
  AMK FR/1("Torque_Output ") -> T_FR/1, Mux/2  "T_FR"
  Read CM Dict17/1 -> AMK RL/3("Torque_limit_pos ")
  Read CM Dict18/1 -> AMK RL/4(Torque_limit_neg)
  Read CM Dict14/1 -> AMK RL/1(Motor_speed_ref_in_RPM)
  AMK RL/1("Torque_Output ") -> T_RL/1, Mux/3  "T_RL"
  Read CM Dict20/1 -> AMK RR/2(Whl_speed_rad_per_sec)
  Read CM Dict22/1 -> AMK RR/3("Torque_limit_pos ")
  Read CM Dict23/1 -> AMK RR/4(Torque_limit_neg)
  Read CM Dict19/1 -> AMK RR/1(Motor_speed_ref_in_RPM)
  AMK RR/1("Torque_Output ") -> T_RR/1, Mux/4  "T_RR"
  Mux/1 -> Gain14/1
  Gain14/1 -> "Eng_Torque "/1, To File--/1
  Read CM Dict4/1 -> Gain4/1
  Read CM Dict3/1 -> Gain6/1
  Read CM Dict5/1 -> Gain7/1
  Read CM Dict6/1 -> Gain8/1
  Read CM Dict8/1 -> Gain3/1, AMK FL/3("Torque_limit_pos ")
  Read CM Dict15/1 -> AMK RL/2(Whl_speed_rad_per_sec)
  Gain3/1 -> Eng_Torque 1/1

== system TV_2018_HIL/CarMaker/Subsystem/Control_System /Output Interface reduce slipratio ==
  Ti_lim : Inport
  MATLAB Function : MATLAB Function  TreatAsAtomicUnit=on
  "Ti_pos " : Outport
  Ti_neg : Outport  Port=2
  wi_setpoints : Outport  Port=3
  wires:
  MATLAB Function/2(Ti_neg) -> Ti_neg/1
  Ti_lim/1 -> MATLAB Function/1(Ti)
  MATLAB Function/1(Ti_pos) -> "Ti_pos "/1
  MATLAB Function/3(wi_setpoints) -> wi_setpoints/1

== system TV_2018_HIL/CarMaker/Subsystem/Control_System /Power Limit Torque Reduction Controller 2018 ==
  note: Hvis enable == 2, input 1 blir passet
      | Hvis Enable == {1,2}, input 3 blir passet
  Ti_lim : Inport
  states : Inport  Port=2
  Bus Creator1 : BusCreator  Inputs=4  OutDataTypeStr=Bus: Ti_lim  NonVirtualBus=on
      settings: InheritFromInputs=off
  Bus Creator2 : BusCreator  Inputs=4  OutDataTypeStr=Bus: Motor_Efficiencies  NonVirtualBus=on
      settings: InheritFromInputs=off
  Delay : Delay  DelayLength=1
  Motorestimates : Subsystem
  "Old powerlimiting " : Subsystem  Commented=on
  Powerlimiting_Control_block : MATLAB Function  TreatAsAtomicUnit=on  SystemSampleTime=0.01
  Scope1 : Scope  NumInputPorts=2
  Scope2 : Scope  NumInputPorts=4
  Scope3 : Scope  NumInputPorts=4
  Scope4 : Scope
  Scope8 : Scope  NumInputPorts=5
  Switch : Switch  Threshold=2
  To Workspace : ToWorkspace  VariableName=Powertest  SaveFormat=Timeseries  SampleTime=-1
  extractPower1 : MATLAB Function  TreatAsAtomicUnit=on
  t_lim : Outport
  Efficiency : Outport  Port=2
  wires:
  states/1 -> Powerlimiting_Control_block/1(states), extractPower1/1(states), "Old powerlimiting "/2(states), Motorestimates/1(states)
  Powerlimiting_Control_block/3(RL) -> Bus Creator1/3, Scope8/3
  Powerlimiting_Control_block/1(FL) -> Scope8/1, Bus Creator1/1
  Powerlimiting_Control_block/4(RR) -> Scope8/4, Bus Creator1/4
  Ti_lim/1 -> "Old powerlimiting "/1(ti_lim), Powerlimiting_Control_block/3(Ti_lim)
  Motorestimates/1(Eff_FL) -> Scope2/1, Bus Creator2/1
  Motorestimates/2(Eff_FR) -> Bus Creator2/2
  Motorestimates/3(Eff_RL) -> Bus Creator2/3
  Motorestimates/4(Eff_RR) -> Bus Creator2/4
  Bus Creator2/1 -> Efficiency/1, Powerlimiting_Control_block/2(Motor_Efficiencies)
  extractPower1/1(power) -> To Workspace/1, Scope1/2
  Powerlimiting_Control_block/6(test1) -> Scope3/1
  Powerlimiting_Control_block/5(state) -> Scope4/1
  Powerlimiting_Control_block/2(FR) -> Bus Creator1/2, Scope8/2
  Bus Creator1/1 -> Delay/1, t_lim/1
  Delay/1 -> Motorestimates/2(Ti_lim)

== system TV_2018_HIL/CarMaker/Subsystem/Control_System /Slip Rate Control  ==
  Ti_ref : Inport
  "States " : Inport  Port=2
  T_req : Inport  Port=3
  Bus Selector : BusSelector  OutputSignals=FL,FR,RL,RR
  Constant : Constant  Value=0
  Index Vector : MultiPortSwitch  DataPortOrder=Zero-based contiguous  Inputs=2  zeroidx=on
  Mux18 : Mux
  SMC Traction Control : Subsystem  Commented=on
  SUM : Subsystem
  Traction Controllers : Subsystem
  tcOutput : Scope
  Ti_lim : Outport
  T_sum_TC : Outport  Port=2
  wires:
  "States "/1 -> Traction Controllers/1(states)
  Ti_ref/1 -> Traction Controllers/2(Ti_ref), Index Vector/2
  Index Vector/1 -> Ti_lim/1
  Constant/1 -> Index Vector/1
  T_req/1 -> Traction Controllers/3(T_requested)
  Mux18/1 -> tcOutput/1
  Bus Selector/1 -> Mux18/1  "<FL>"
  Bus Selector/2 -> Mux18/2  "<FR>"
  Bus Selector/3 -> Mux18/3  "<RL>"
  Bus Selector/4 -> Mux18/4  "<RR>"
  Traction Controllers/1(Ti_SR) -> SUM/1(In1), Bus Selector/1, Index Vector/3
  SUM/1(Out1) -> T_sum_TC/1

== system TV_2018_HIL/CarMaker/Subsystem/Control_System /Subsystem ==
  In1 : Inport
  In2 : Inport  Port=2
  In3 : Inport  Port=3
  In4 : Inport  Port=4
  In5 : Inport  Port=5
  In6 : Inport  Port=6
  In7 : Inport  Port=7
  In8 : Inport  Port=8
  In9 : Inport  Port=9
  In10 : Inport  Port=10
  In11 : Inport  Port=11
  In12 : Inport  Port=12
  In13 : Inport  Port=13
  In14 : Inport  Port=14
  In15 : Inport  Port=15
  In16 : Inport  Port=16
  In17 : Inport  Port=17
  In18 : Inport  Port=18
  In19 : Inport  Port=19
  2016 adapted : Subsystem  Commented=on
  OutputTelemetri : MATLAB Function  Commented=on  TreatAsAtomicUnit=on
  Torque allocation 2016 : Subsystem  Commented=on
  Torque allocation 2017 : Subsystem  Commented=on
  Torque allocation QP- : Subsystem  Commented=on
  Torque allocation QP-1 : Subsystem  Commented=on
  Out1 : Outport
  Out2 : Outport  Port=2
  Out3 : Outport  Port=3
  Out4 : Outport  Port=4
  Out5 : Outport  Port=5
  Out6 : Outport  Port=6
  Out7 : Outport  Port=7
  Out8 : Outport  Port=8
  Out9 : Outport  Port=9
  Out10 : Outport  Port=10
  Out11 : Outport  Port=11
  Out12 : Outport  Port=12
  Out13 : Outport  Port=13
  Out14 : Outport  Port=14
  Out15 : Outport  Port=15
  Out16 : Outport  Port=16
  Out17 : Outport  Port=17
  Out18 : Outport  Port=18
  Out19 : Outport  Port=19
  Out20 : Outport  Port=20
  Out21 : Outport  Port=21
  Out22 : Outport  Port=22
  Out23 : Outport  Port=23
  Out24 : Outport  Port=24
  wires:
  2016 adapted/3(saturated_constraints) -> Out12/1
  In4/1 -> Torque allocation QP-/2(T_req)
  Torque allocation QP-/1("Mz_allocated ") -> Out1/1
  Torque allocation QP-/4(max_motor_torque) -> Out6/1
  In17/1 -> Torque allocation QP-1/2(T_req)
  In19/1 -> Torque allocation QP-1/3("States ")
  Torque allocation QP-1/2(Ti_lim) -> Out18/1
  Torque allocation QP-1/4(max_motor_torque) -> Out21/1
  2016 adapted/2(Ti_lim) -> Out10/1
  2016 adapted/1("Mz_allocated ") -> Out9/1
  In1/1 -> Torque allocation 2016/1(Mz_ref)
  In3/1 -> Torque allocation 2016/2(T_req)
  Torque allocation QP-/5(active_constraints) -> Out8/1
  In5/1 -> Torque allocation 2016/3("States ")
  Torque allocation QP-1/3(saturated_constraints) -> Out20/1
  2016 adapted/4(Max_motor_torque) -> Out13/1
  In6/1 -> Torque allocation QP-/3("States ")
  Torque allocation QP-1/5(active_constraints) -> Out23/1
  Torque allocation 2016/1(Ti_lim) -> Out2/1
  Torque allocation QP-/2(Ti_lim) -> Out3/1
  Torque allocation QP-/3(saturated_constraints) -> Out5/1
  In15/1 -> Torque allocation QP-1/1(Mz_ref)
  Torque allocation QP-1/1("Mz_allocated ") -> Out16/1
  In12/1 -> 2016 adapted/3("States ")
  In8/1 -> 2016 adapted/1(Mz_ref)
  In2/1 -> Torque allocation QP-/1(Mz_ref)
  2016 adapted/5(active_constraints) -> Out14/1
  In10/1 -> 2016 adapted/2(T_req)
  Torque allocation 2017/1("Mz_allocated ") -> Out15/1
  In9/1 -> OutputTelemetri/2(T_req)
  In18/1 -> Torque allocation 2017/3("States ")
  Torque allocation 2017/5(active_constraints) -> Out24/1
  In7/1 -> OutputTelemetri/1(states)
  In11/1 -> OutputTelemetri/3(r_ref)
  Torque allocation 2017/3(saturated_constraints) -> Out19/1
  Torque allocation 2017/2(Ti_lim) -> Out17/1
  In16/1 -> Torque allocation 2017/2(T_req)
  Torque allocation 2016/2("Mz_error ") -> Out4/1
  In14/1 -> Torque allocation 2017/1(Mz_ref)
  Torque allocation 2017/4(max_motor_torque) -> Out22/1
  Torque allocation 2016/3(Max_motor_torque_i) -> Out7/1
  In13/1 -> OutputTelemetri/4(Mz_ref_to_telemetry)
  OutputTelemetri/1(OutputTelemetri_control) -> Out11/1

== system TV_2018_HIL/CarMaker/Subsystem/Control_System /TA 2017 ==
  Mz_ref : Inport
  T_req : Inport  Port=2
  "States " : Inport  Port=3
  T_req1 : Inport  Port=4
  Bus Selector1 : BusSelector  OutputSignals=mmt_FL,mmt_FR,mmt_RL,mmt_RR
  Bus Selector2 : BusSelector  OutputSignals=mmt_FL,mmt_FR,mmt_RL,mmt_RR
  Bus Selector3 : BusSelector  OutputSignals=FL,FR,RL,RR
  Bus Selector6 : BusSelector  OutputSignals=FL,FR,RL,RR
  Friction Torque Limits : Scope
  Mux{1..4,7} (5 alike) : Mux
  Mz : Scope
  Mz1 : Scope
  "Slip handling (Traction Control) " : Subsystem
  SlipScalingFactor : Scope
  Ti_Lim_TA : Scope
  Ti_max : Scope
  Torque lim Slip : Scope
  TorqueAllocation : MATLAB Function  TreatAsAtomicUnit=on
  TorqueLimFZ : Scope
  "max combined tire torque based on (Fz, SA,mu) " : MATLAB Function  TreatAsAtomicUnit=on
  "max long tire torque based on (FZ , mu)" : MATLAB Function  TreatAsAtomicUnit=on
  "max torque " : MATLAB Function  TreatAsAtomicUnit=on
  required torque : Scope  NumInputPorts=4
  "Mz_error " : Outport
  Ti_lim : Outport  Port=2
  pow_red : Outport  Port=3
  max_motor_torque : Outport  Port=4
  active_constraints : Outport  Port=5
  overiterate 1 : Outport  Port=6
  wires:
  Mux1/1 -> Mz/1
  TorqueAllocation/4(Mz_allocated) -> required torque/4, Mux1/2  "Mz_all"
  TorqueAllocation/2(pow_red) -> pow_red/1, Ti_max/1
  Mz_ref/1 -> required torque/2, Mux1/3, TorqueAllocation/1(Mz_ref)  "Mz_ref"
  "States "/1 -> [states], TorqueAllocation/3(states)
  "max torque "/2(active_constraints) -> [active_constraints]
  "max long tire torque based on (FZ , mu)"/1(maxMotorTorque) -> Bus Selector2/1, "max torque "/1(mu_lim)
  [maxMotorTorque] -> max_motor_torque/1
  [active_constraints] -> active_constraints/1
  "max torque "/1(maxMotorTorque) -> [maxMotorTorque]
  [maxMotorTorque] -> TorqueAllocation/4(maxMotorTorque)
  TorqueAllocation/3(Mz_error) -> required torque/3, Mux1/1, "Mz_error "/1  "Mz_error"
  "max torque "/3(friction_limits) -> Friction Torque Limits/1, [friction_torque_limits]
  [friction_torque_limits] -> TorqueAllocation/5(friction_limit_torques)
  TorqueAllocation/5(overiterate) -> overiterate 1/1
  "max combined tire torque based on (Fz, SA,mu) "/1(maxMotorTorque) -> "max torque "/4(mot_temp_lim), "max torque "/3(inv_temp_lim), "max torque "/2(SA_lim), Bus Selector1/1
  [states] -> "Slip handling (Traction Control) "/1(Sensors), "max long tire torque based on (FZ , mu)"/1(states), "max combined tire torque based on (Fz, SA,mu) "/1(states)
  Bus Selector6/1 -> Mux7/1  "<FL>"
  Bus Selector6/2 -> Mux7/2  "<FR>"
  Bus Selector6/3 -> Mux7/3  "<RL>"
  Bus Selector6/4 -> Mux7/4  "<RR>"
  TorqueAllocation/1(Ti_lim) -> Bus Selector6/1, Ti_lim/1
  Mux7/1 -> Ti_Lim_TA/1
  Bus Selector1/1 -> Mux2/1  "<mmt_FL>"
  Bus Selector1/2 -> Mux2/2  "<mmt_FR>"
  Bus Selector1/3 -> Mux2/3  "<mmt_RL>"
  Bus Selector1/4 -> Mux2/4  "<mmt_RR>"
  Mux2/1 -> Torque lim Slip/1
  Bus Selector2/1 -> Mux3/1  "<mmt_FL>"
  Bus Selector2/2 -> Mux3/2  "<mmt_FR>"
  Bus Selector2/3 -> Mux3/3  "<mmt_RL>"
  Bus Selector2/4 -> Mux3/4  "<mmt_RR>"
  Mux3/1 -> TorqueLimFZ/1
  Bus Selector3/1 -> Mux4/1  "<FL>"
  Bus Selector3/2 -> Mux4/2  "<FR>"
  Bus Selector3/3 -> Mux4/3  "<RL>"
  Bus Selector3/4 -> Mux4/4  "<RR>"
  Mux4/1 -> SlipScalingFactor/1
  "Slip handling (Traction Control) "/1(slipScalingFactors) -> "max torque "/5(slipScalingFactors), Bus Selector3/1
  T_req/1 -> required torque/1, Mux1/4, TorqueAllocation/2(T_req)
  ? -> Mz1/1
  T_req1/1 -> TorqueAllocation/6(Motoreff)

== system TV_2018_HIL/CarMaker/Subsystem/Control_System /Yaw_rate_Mz_generator ==
  Mz_error : Inport
  States : Inport  Port=2
  Enable/disable : Constant  Value=yawRateControl.method
  "Mz_1 , Mz_2" : Scope  NumInputPorts=2
  Switch : Switch  Threshold=1.5
  Switch1 : Switch  Criteria=u2 > Threshold
  "Yaw Rate Controller " : Subsystem
  Yaw Rate Generator : Subsystem
  Mz_Ref : Outport
  r_ref : Outport  Port=2
  wires:
  "Yaw Rate Controller "/3(Mz_ref) -> "Mz_1 , Mz_2"/1, Switch/1
  "Yaw Rate Controller "/1("r_ref ") -> r_ref/1  "r_ref"
  "Yaw Rate Controller "/4(Mz_ref_to_telemetry) -> Switch1/1
  Yaw Rate Generator/1(Mz_ref) -> "Mz_1 , Mz_2"/2, Switch/3
  Yaw Rate Generator/2(Mz_ref_to_telemetry) -> Switch1/3
  States/1 -> "Yaw Rate Controller "/2(States), Yaw Rate Generator/1(States)
  Mz_error/1 -> "Yaw Rate Controller "/1("Mz_error ")
  Switch/1 -> Mz_Ref/1
  Switch1/1 -> [Mz_ref_tt]
  Enable/disable/1 -> Switch1/2, Switch/2

== system TV_2018_HIL/CarMaker/Subsystem/Debug Information /Extract and scale to deg compare to CM output in individual error ==
  SA_CM : Inport
  In1 : Inport  Port=2
  Bus Selector1 : BusSelector  OutputSignals=FL,FR,RL,RR
  Demux : Demux
  Rate Transition2 : RateTransition  OutPortSampleTime=0.001
  SA  estimate : Scope  NumInputPorts=4
  Sum{,1..3} (4 alike) : Sum  Inputs=|-+
  r2d{,1..3} (4 alike) : simulink_extras/Transformations/Radians to Degrees
  FL : Outport
  FR : Outport  Port=2
  RL : Outport  Port=3
  RR : Outport  Port=4
  wires:
  SA_CM/1 -> Demux/1
  Demux/1 -> Sum/1
  r2d/1 -> Sum/2, SA  estimate/1
  Demux/2 -> Sum1/1
  r2d1/1 -> Sum1/2, SA  estimate/2
  Demux/3 -> Sum2/1
  r2d2/1 -> Sum2/2, SA  estimate/3
  Demux/4 -> Sum3/1
  r2d3/1 -> SA  estimate/4, Sum3/2
  Sum/1 -> FL/1
  Sum1/1 -> FR/1
  Sum2/1 -> RL/1
  Sum3/1 -> RR/1
  In1/1 -> Rate Transition2/1
  Bus Selector1/1 -> r2d/1  "<FL>"
  Bus Selector1/2 -> r2d1/1  "<FR>"
  Bus Selector1/3 -> r2d2/1  "<RL>"
  Bus Selector1/4 -> r2d3/1  "<RR>"
  Rate Transition2/1 -> Bus Selector1/1

== system TV_2018_HIL/CarMaker/Subsystem/Debug Information /Extract and scale to deg compare to CM output in individual error1 ==
  SA_CM : Inport
  In1 : Inport  Port=2
  Bus Selector1 : BusSelector  OutputSignals=SR_FL,SR_FR,SR_RL,SR_RR
  Demux : Demux
  Rate Transition2 : RateTransition  OutPortSampleTime=0.001
  SR  estimate : Scope  NumInputPorts=4
  Sum{,1..3} (4 alike) : Sum  Inputs=|-+
  r2d{,1..3} (4 alike) : simulink_extras/Transformations/Radians to Degrees  Commented=on
  FL : Outport
  FR : Outport  Port=2
  RL : Outport  Port=3
  RR : Outport  Port=4
  wires:
  SA_CM/1 -> Demux/1
  Demux/1 -> Sum/1
  Demux/2 -> Sum1/1
  Demux/3 -> Sum2/1
  Demux/4 -> Sum3/1
  Sum/1 -> FL/1
  Sum1/1 -> FR/1
  Sum2/1 -> RL/1
  Sum3/1 -> RR/1
  In1/1 -> Rate Transition2/1
  Bus Selector1/1 -> Sum/2, SR  estimate/1  "<SR_FL>"
  Bus Selector1/2 -> Sum1/2, SR  estimate/2  "<SR_FR>"
  Bus Selector1/3 -> Sum2/2, SR  estimate/3  "<SR_RL>"
  Bus Selector1/4 -> SR  estimate/4, Sum3/2  "<SR_RR>"
  Rate Transition2/1 -> Bus Selector1/1

== system TV_2018_HIL/CarMaker/Subsystem/Debug Information /Fz_Estimation ==
  sensors : Inport
  v_x : Inport  Port=2
  Bus Selector : BusSelector  OutputSignals=damper_rate_FL,damper_rate_FR,damper_rate_RL,damper_rate_RR
  Bus Selector1 : BusSelector  OutputSignals=FL,FR,RL,RR
  Bus Selector2 : BusSelector  OutputSignals=FL,FR,RL,RR
  Constant : Constant  Value=settings.select_Fz_est_method
  DamperRateLookup : Lookup_n-D  NumberOfTableDimensions=1  BreakpointsForDimension1=car_params.damper_table_breakpoint;  Table=car_params.damper_pull_push_values_front;  ExtrapMethod=Clip  UseLastTableValue=on  InternalRulePriority=Speed  RndMeth=Simplest  InputSameDT=on
  DamperRateLookup1 : Lookup_n-D  NumberOfTableDimensions=1  BreakpointsForDimension1=car_params.damper_table_breakpoint;  Table=car_params.damper_pull_push_values_front;  ExtrapMethod=Clip  UseLastTableValue=on  InternalRulePriority=Speed  RndMeth=Simplest  InputSameDT=on
  DamperRateLookup2 : Lookup_n-D  NumberOfTableDimensions=1  BreakpointsForDimension1=car_params.damper_table_breakpoint;  Table=car_params.damper_pull_push_values_rear;  ExtrapMethod=Clip  UseLastTableValue=on  InternalRulePriority=Speed  RndMeth=Simplest  InputSameDT=on
  DamperRateLookup3 : Lookup_n-D  NumberOfTableDimensions=1  BreakpointsForDimension1=car_params.damper_table_breakpoint;  Table=car_params.damper_pull_push_values_rear;  ExtrapMethod=Clip  UseLastTableValue=on  InternalRulePriority=Speed  RndMeth=Simplest  InputSameDT=on
  DamperRateLookup4 : Lookup_n-D  Commented=on  NumberOfTableDimensions=1  BreakpointsForDimension1=single([-200,0,200]);  Table=single([-500,0,500]);  ExtrapMethod=Clip  UseLastTableValue=on  InternalRulePriority=Speed  RndMeth=Simplest  InputSameDT=on
  DamperRateLookup5 : Lookup_n-D  Commented=on  NumberOfTableDimensions=1  BreakpointsForDimension1=single([-200,0,200]);  Table=single([-500,0,500]);  ExtrapMethod=Clip  UseLastTableValue=on  InternalRulePriority=Speed  RndMeth=Simplest  InputSameDT=on
  FzEstDamper : MATLAB Function  TreatAsAtomicUnit=on
  FzEstDamper 2016 : MATLAB Function  Commented=on  TreatAsAtomicUnit=on
  FzEstLoadTransfer : MATLAB Function  TreatAsAtomicUnit=on
  Index Vector : MultiPortSwitch  Inputs=2
  Scope : Scope  NumInputPorts=4
  Scope1 : Scope  NumInputPorts=4
  Fz_est : Outport
  Fz_LoadTransfer_est : Outport  Port=2
  Fz_damper_est : Outport  Port=3
  alfa_r : Outport  Port=4
  wires:
  sensors/1 -> FzEstLoadTransfer/1(sensor), FzEstDamper/1(sensors), Bus Selector/1
  DamperRateLookup/1 -> FzEstDamper/2(Fz_damp_FL)  "Fz_damp_FL"
  Bus Selector/1 -> DamperRateLookup/1  "<damper_rate_FL>"
  Bus Selector/2 -> DamperRateLookup1/1  "<damper_rate_FR>"
  Bus Selector/3 -> DamperRateLookup2/1  "<damper_rate_RL>"
  Bus Selector/4 -> DamperRateLookup3/1  "<damper_rate_RR>"
  DamperRateLookup1/1 -> FzEstDamper/3(Fz_damp_FR)
  DamperRateLookup2/1 -> FzEstDamper/4(Fz_damp_RL)
  DamperRateLookup3/1 -> FzEstDamper/5(Fz_damp_RR)
  Index Vector/1 -> Fz_est/1
  v_x/1 -> FzEstLoadTransfer/2(vx)
  FzEstDamper/2(alfa_r) -> alfa_r/1
  Bus Selector1/2 -> Scope/2  "<FR>"
  Bus Selector1/1 -> Scope/1  "<FL>"
  Bus Selector1/3 -> Scope/3  "<RL>"
  Bus Selector1/4 -> Scope/4  "<RR>"
  Constant/1 -> Index Vector/1
  FzEstLoadTransfer/1(Fz_loadTransfer_est) -> Bus Selector2/1, Fz_LoadTransfer_est/1, Index Vector/2
  Bus Selector2/2 -> Scope1/2  "<FR>"
  Bus Selector2/1 -> Scope1/1  "<FL>"
  Bus Selector2/3 -> Scope1/3  "<RL>"
  Bus Selector2/4 -> Scope1/4  "<RR>"
  FzEstDamper/1(Fz_damper_est) -> Index Vector/3, Bus Selector1/1, Fz_damper_est/1
  DamperRateLookup4/1 -> FzEstDamper 2016/3(Fz_damp_FR)
  DamperRateLookup5/1 -> FzEstDamper 2016/4(Fz_damp_RL)
